simulink model "EPS_Phase_Shift_Control_Model_No_DeadTimeV1_0"  (R2016b)
settings: Solver=VariableStepAuto  StartTime=0.0  StopTime=5/100000  MaxStep=1e-9  RelTol=1e-3
libraries: simulink_extras x4
settings Model: Creator=whl14  LastModifiedBy=whl14

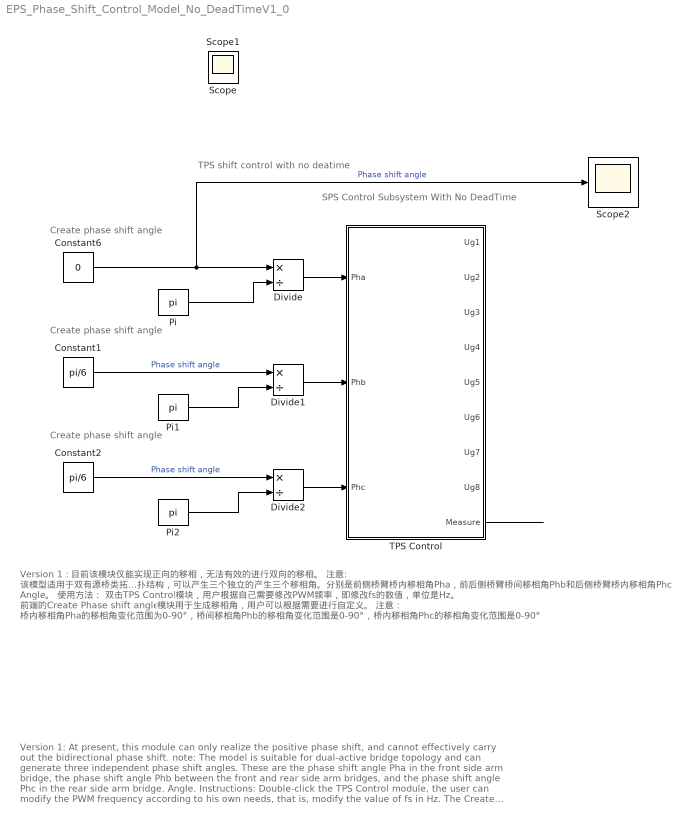
== system EPS_Phase_Shift_Control_Model_No_DeadTimeV1_0 ==
  note: TPS shift control with no deatime
  note: Version 1:
      | At present, this module can only realize the positive phase shift, and cannot effectively carry out the bidirectional phase shift.
      | note:
      | The model is suitable for dual-active bridge topology and can generate three independent phase shift angles. These are the phase shift angle Pha in the front side arm bridge, the phase shift angle Phb between the front and rear side arm bridges, and the phase shift angle Phc in the rear side arm bridge.
      | Angle.
      | Instructions:
      | Double-click the TPS Control module, the user can modify the PWM frequency according to his own needs, that is, modify the value of fs in Hz.
      | The Create Phase shift angle module at the front end is used to generate the phase shift angle, and the user can customize it as needed.
      | note:
      | The phase shift angle of the bridge phase shift angle Pha varies from 0-90°, the phase shift angle of the inter-bridge phase shift angle Phb varies from 0-90°, and the phase shift angle of the phase shift angle Phc within the bridge varies from 0 -90°
  note: Version 1 :
      | 目前该模块仅能实现正向的移相，无法有效的进行双向的移相。
      | 注意:
      | 该模型适用于双有源桥类拓扑结构，可以产生三个独立的产生三个移相角。分别是前侧桥臂桥内移相角Pha，前后侧桥臂桥间移相角Phb和后侧桥臂桥内移相角Phc
      | Angle。
      | 使用方法：
      | 双击TPS Control模块，用户根据自己需要修改PWM频率，即修改fs的数值，单位是Hz。
      | 前端的Create Phase shift angle模块用于生成移相角，用户可以根据需要进行自定义。
      | 注意：
      | 桥内移相角Pha的移相角变化范围为0-90°，桥间移相角Phb的移相角变化范围是0-90°，桥内移相角Phc的移相角变化范围是0-90°
  note: Create phase shift angle
  note: SPS Control Subsystem With No DeadTime
  note: Create phase shift angle
  note: Create phase shift angle
  Constant1 : Constant  Value=pi/6
  Constant2 : Constant  Value=pi/6
  Constant6 : Constant  Value=0
  Divide : Product  Inputs=*/
  Divide1 : Product  Inputs=*/
  Divide2 : Product  Inputs=*/
  Pi : Constant  Value=pi
  Pi1 : Constant  Value=pi
  Pi2 : Constant  Value=pi
  Scope2 : Scope
  TPS Control : Subsystem  mask(SPS Control SubModel description){fs=100000}
      mask help:
      | Define the frequency about the PWM, double clik the subsystem 'SPS Control' and change the value about the fs
      |
      | The input signal is a phase shift angle, which can be defined by the user as required
      mask Display:
      | color('red');
      | text(20,170,'Phase Shift Control');
      | color('Blue');
      | disp('TPS Control');
  Scope : Scope
  Scope1 : Scope
  wires:
  Constant6/1 -> Scope2/1, Divide/1  "Phase shift angle"
  Pi/1 -> Divide/2
  TPS Control/9(Measure) -> ?
  Constant1/1 -> Divide1/1  "Phase shift angle"
  Pi1/1 -> Divide1/2
  Constant2/1 -> Divide2/1  "Phase shift angle"
  Pi2/1 -> Divide2/2
  Divide2/1 -> TPS Control/3(Phc)
  Divide1/1 -> TPS Control/2(Phb)
  Divide/1 -> TPS Control/1(Pha)

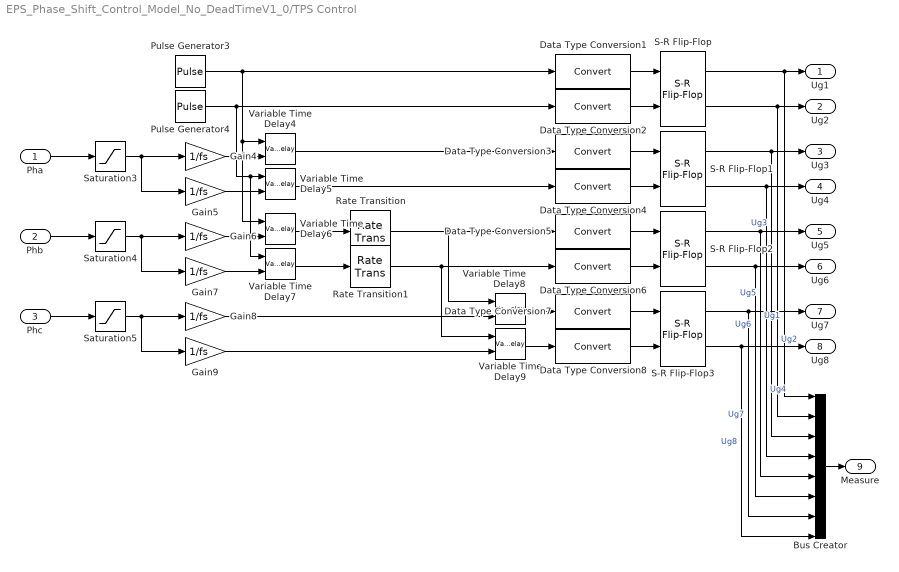
== system EPS_Phase_Shift_Control_Model_No_DeadTimeV1_0/TPS Control ==
  Pha : Inport
  Phb : Inport  Port=2
  Phc : Inport  Port=3
  Bus Creator : BusCreator  Inputs=8
  Data Type Conversion{1..8} (8 alike) : DataTypeConversion
  Gain{4..9} (6 alike) : Gain  Gain=1/fs
  Pulse Generator3 : DiscretePulseGenerator  PulseType=Time based  Period=1/(1*fs)  PulseWidth=50  VectorParams1D=off
  Pulse Generator4 : DiscretePulseGenerator  PulseType=Time based  Period=1/(1*fs)  PulseWidth=50  PhaseDelay=0.5/fs  VectorParams1D=off
  Rate Transition : RateTransition
  Rate Transition1 : RateTransition
  S-R Flip-Flop{,1..3} (4 alike) : simulink_extras/Flip Flops/S-R Flip-Flop  initial_condition=0
  Saturation3 : Saturate  LowerLimit=0
  Saturation4 : Saturate  LowerLimit=0
  Saturation5 : Saturate  UpperLimit=1  LowerLimit=0
  Variable Time Delay{4..9} (6 alike) : VariableTransportDelay  MaximumDelay=10  ZeroDelay=on
  Ug1 : Outport
  Ug2 : Outport  Port=2
  Ug3 : Outport  Port=3
  Ug4 : Outport  Port=4
  Ug5 : Outport  Port=5
  Ug6 : Outport  Port=6
  Ug7 : Outport  Port=7
  Ug8 : Outport  Port=8
  Measure : Outport  Port=9
  wires:
  Bus Creator/1 -> Measure/1
  Data Type Conversion1/1 -> S-R Flip-Flop/1
  Data Type Conversion2/1 -> S-R Flip-Flop/2
  Gain4/1 -> Variable Time Delay4/2
  Pha/1 -> Saturation3/1
  Variable Time Delay4/1 -> Data Type Conversion3/1
  Gain5/1 -> Variable Time Delay5/2
  Saturation3/1 -> Gain5/1, Gain4/1
  Variable Time Delay5/1 -> Data Type Conversion4/1
  S-R Flip-Flop/1 -> Bus Creator/1, Ug1/1  "Ug1"
  S-R Flip-Flop/2 -> Bus Creator/2, Ug2/1  "Ug2"
  S-R Flip-Flop1/1 -> Ug3/1, Bus Creator/3  "Ug3"
  S-R Flip-Flop1/2 -> Bus Creator/4, Ug4/1  "Ug4"
  Data Type Conversion3/1 -> S-R Flip-Flop1/1
  Data Type Conversion4/1 -> S-R Flip-Flop1/2
  Pulse Generator3/1 -> Variable Time Delay6/1, Variable Time Delay4/1, Data Type Conversion1/1
  Pulse Generator4/1 -> Variable Time Delay7/1, Variable Time Delay5/1, Data Type Conversion2/1
  Gain6/1 -> Variable Time Delay6/2
  Phb/1 -> Saturation4/1
  Gain7/1 -> Variable Time Delay7/2
  Saturation4/1 -> Gain7/1, Gain6/1
  S-R Flip-Flop2/1 -> Bus Creator/5, Ug5/1  "Ug5"
  S-R Flip-Flop2/2 -> Bus Creator/6, Ug6/1  "Ug6"
  Data Type Conversion5/1 -> S-R Flip-Flop2/1
  Data Type Conversion6/1 -> S-R Flip-Flop2/2
  Variable Time Delay6/1 -> Rate Transition/1
  Variable Time Delay7/1 -> Rate Transition1/1
  Gain8/1 -> Variable Time Delay8/2
  Phc/1 -> Saturation5/1
  Variable Time Delay8/1 -> Data Type Conversion7/1
  Gain9/1 -> Variable Time Delay9/2
  Saturation5/1 -> Gain9/1, Gain8/1
  Variable Time Delay9/1 -> Data Type Conversion8/1
  S-R Flip-Flop3/1 -> Bus Creator/7, Ug7/1  "Ug7"
  S-R Flip-Flop3/2 -> Bus Creator/8, Ug8/1  "Ug8"
  Data Type Conversion7/1 -> S-R Flip-Flop3/1
  Data Type Conversion8/1 -> S-R Flip-Flop3/2
  Rate Transition/1 -> Data Type Conversion5/1, Variable Time Delay8/1
  Rate Transition1/1 -> Data Type Conversion6/1, Variable Time Delay9/1
